simulink model "ssv_ssv_control"  (R2024a)
settings: Solver=VariableStepAuto  StartTime=0.0  StopTime=60.0  RelTol=1e-3
settings Model: Creator=MARTENAG  LastModifiedBy=MARTENAG

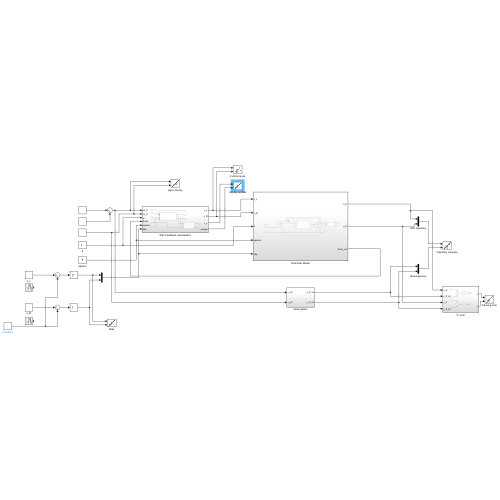
[thumbnail: Simulink's stored preview of the top-level diagram]
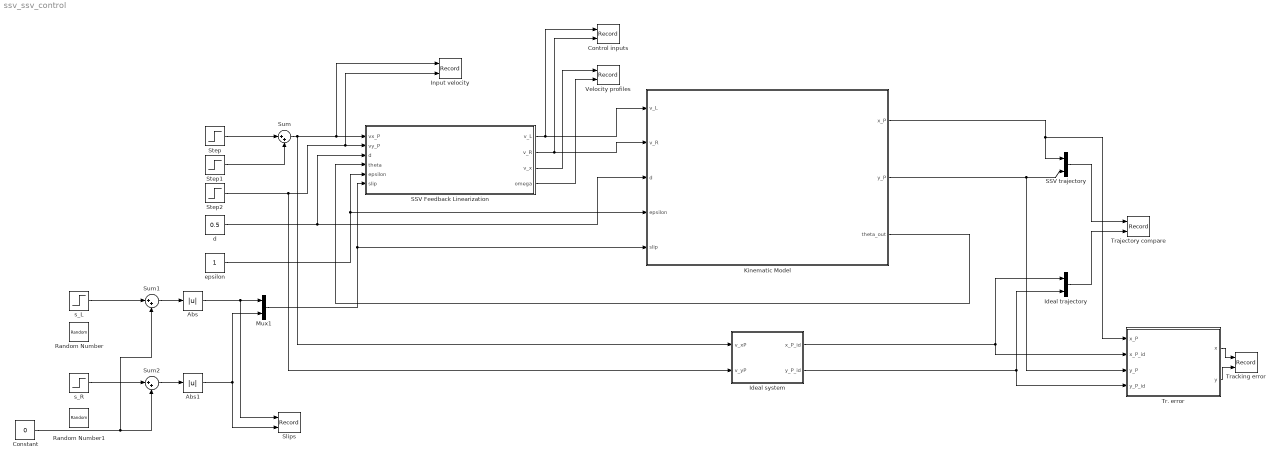
== system ssv_ssv_control ==
  Abs : Abs  SaturateOnIntegerOverflow=off
  Abs1 : Abs  SaturateOnIntegerOverflow=off
  Constant : Constant  Value=0
  Control inputs : Record  FileSettingsInternal="{\"entries\":[{\"content\":{\"excelSettings\":{\"content\":{},\"type\":\"Streamout.ExcelSettings\"}},\"type\":\"Streamout.FileSettingStorage\",\"uuid\":\"\"}],\"packageUris\":[\"http:\\/\\/schema.mathworks.com\\/mf0\\/streamout_blocks\\/R2020a\"],\"version\":\"1.0\"}"  Layout=[1 1]  SignalsInternal="{\"entries\":[{\"content\":{\"signals\":[{\"content\":{\"blockPath\":[],\"dimensions\":[1],\"domain\":\"\",\"lineColor\":\"#a2142f\",\"plots\":[ 1 ],\"port\":1,\"sid\":[\"\"],\"signalID\":1,\"signalName\":\"v_L\"},\"type\":\"RecordBlkView.Signal\",\"uuid\":\"\"},{\"content\":{\"blockPath\":[],\"dimensions\":[1],\"domain\":\"\",\"lineColor\":\"#139fff\",\"plots\":[ 1 ],\"port\":2,\"sid\":[\"\"],\"signalID\":2,\"signalName\":\"v_R\"},\"type\":\"RecordBlkView.Signal\",\"uuid\":\"\"}]},\"type\":\"RecordBlkView.InputSignals\",\"uuid\":\"\"}],\"packageUris\":[\"http:\\/\\/schema.mathworks.com\\/mf0\\/streamout_blocks\\/R2020a\"],\"version\":\"1.0\"}"  VisualizationBindings="{\"sparklinesplugin\":{\"info\":[{\"bindingParametersList\":[],\"subplotID\":1}]}}"  CompatibilityTag=XY
  Ideal system : Subsystem
  Ideal trajectory : Mux  Inputs=2
  Input velocity : Record  FileSettingsInternal="{\"entries\":[{\"content\":{\"excelSettings\":{\"content\":{},\"type\":\"Streamout.ExcelSettings\"}},\"type\":\"Streamout.FileSettingStorage\",\"uuid\":\"\"}],\"packageUris\":[\"http:\\/\\/schema.mathworks.com\\/mf0\\/streamout_blocks\\/R2020a\"],\"version\":\"1.0\"}"  Layout=[1 1]  SignalsInternal="{\"entries\":[{\"content\":{\"signals\":[{\"content\":{\"blockPath\":[],\"dimensions\":[1],\"domain\":\"\",\"lineColor\":\"#a2142f\",\"plots\":[ 1 ],\"port\":1,\"sid\":[\"\"],\"signalID\":1,\"signalName\":\"Sum\"},\"type\":\"RecordBlkView.Signal\",\"uuid\":\"\"},{\"content\":{\"blockPath\":[],\"dimensions\":[1],\"domain\":\"\",\"lineColor\":\"#139fff\",\"plots\":[ 1 ],\"port\":2,\"sid\":[\"\"],\"signalID\":2,\"signalName\":\"Step2\"},\"type\":\"RecordBlkView.Signal\",\"uuid\":\"\"}]},\"type\":\"RecordBlkView.InputSignals\",\"uuid\":\"\"}],\"packageUris\":[\"http:\\/\\/schema.mathworks.com\\/mf0\\/streamout_blocks\\/R2020a\"],\"version\":\"1.0\"}"  CompatibilityTag=XY
  Kinematic Model : Subsystem
  Mux1 : Mux  Inputs=2
  Random Number : RandomNumber  Mean=0.08  Variance=0.01  SampleTime=0.1
  Random Number1 : RandomNumber  Mean=0.08  Variance=0.01  SampleTime=0.1
  SSV Feedback Linearization : Subsystem
  SSV trajectory : Mux  Inputs=2
  Slips : Record  FileSettingsInternal="{\"entries\":[{\"content\":{\"excelSettings\":{\"content\":{},\"type\":\"Streamout.ExcelSettings\"}},\"type\":\"Streamout.FileSettingStorage\",\"uuid\":\"\"}],\"packageUris\":[\"http:\\/\\/schema.mathworks.com\\/mf0\\/streamout_blocks\\/R2020a\"],\"version\":\"1.0\"}"  Layout=[1 1]  SignalsInternal="{\"entries\":[{\"content\":{\"signals\":[{\"content\":{\"blockPath\":[],\"dimensions\":[1],\"domain\":\"\",\"lineColor\":\"#77ac30\",\"lineWidth\":2,\"plots\":[ 1 ],\"port\":1,\"sid\":[\"\"],\"signalID\":1,\"signalName\":\"Abs\"},\"type\":\"RecordBlkView.Signal\",\"uuid\":\"\"},{\"content\":{\"blockPath\":[],\"dimensions\":[1],\"domain\":\"\",\"lineColor\":\"#4dbeee\",\"lineWidth\":2,\"plots\":[ 1 ],\"port\":2,\"sid\":[\"\"],\"signalID\":2,\"signalName\":\"Abs1\"},\"type\":\"RecordBlkView.Signal\",\"uuid\":\"\"}]},\"type\":\"RecordBlkView.InputSignals\",\"uuid\":\"\"}],\"packageUris\":[\"http:\\/\\/schema.mathworks.com\\/mf0\\/streamout_blocks\\/R2020a\"],\"version\":\"1.0\"}"  VisualizationBindings="{\"sparklinesplugin\":{\"info\":[{\"bindingParametersList\":[],\"subplotID\":1}]}}"  CompatibilityTag=XY
  Step : Step  SampleTime=0
  Step1 : Step  Time=5  SampleTime=0
  Step2 : Step  Time=10  SampleTime=0
  Sum : Sum  Inputs=|++
  Sum1 : Sum  Inputs=|++
  Sum2 : Sum  Inputs=|++
  Tr. error : Subsystem
  Tracking error : Record  FileSettingsInternal="{\"entries\":[{\"content\":{\"excelSettings\":{\"content\":{},\"type\":\"Streamout.ExcelSettings\"}},\"type\":\"Streamout.FileSettingStorage\",\"uuid\":\"\"}],\"packageUris\":[\"http:\\/\\/schema.mathworks.com\\/mf0\\/streamout_blocks\\/R2020a\"],\"version\":\"1.0\"}"  Layout=[1 1]  SignalsInternal="{\"entries\":[{\"content\":{\"signals\":[{\"content\":{\"blockPath\":[],\"dimensions\":[1],\"domain\":\"\",\"lineColor\":\"#fe330a\",\"lineWidth\":2,\"plots\":[ 1 ],\"port\":1,\"sid\":[\"\"],\"signalID\":1,\"signalName\":\"Tr. error:1\"},\"type\":\"RecordBlkView.Signal\",\"uuid\":\"\"},{\"content\":{\"blockPath\":[],\"dimensions\":[1],\"domain\":\"\",\"lineColor\":\"#22b573\",\"lineWidth\":2,\"plots\":[ 1 ],\"port\":2,\"sid\":[\"\"],\"signalID\":2,\"signalName\":\"Tr. error:2\"},\"type\":\"RecordBlkView.Signal\",\"uuid\":\"\"}]},\"type\":\"RecordBlkView.InputSignals\",\"uuid\":\"\"}],\"packageUris\":[\"http:\\/\\/schema.mathworks.com\\/mf0\\/streamout_blocks\\/R2020a\"],\"version\":\"1.0\"}"  VisualizationBindings="{\"sparklinesplugin\":{\"info\":[{\"bindingParametersList\":[],\"subplotID\":1}]}}"  CompatibilityTag=XY
  Trajectory compare : Record  FileSettingsInternal="{\"entries\":[{\"content\":{\"excelSettings\":{\"content\":{},\"type\":\"Streamout.ExcelSettings\"}},\"type\":\"Streamout.FileSettingStorage\",\"uuid\":\"\"}],\"packageUris\":[\"http:\\/\\/schema.mathworks.com\\/mf0\\/streamout_blocks\\/R2020a\"],\"version\":\"1.0\"}"  Layout=[1 1]  SignalsInternal="{\"entries\":[{\"content\":{\"signals\":[{\"content\":{\"blockPath\":[],\"dimensions\":[2],\"domain\":\"\",\"hasChildren\":true,\"lineColor\":\"#77ac30\",\"lineWidth\":2,\"port\":1,\"sid\":[\"\"],\"signalID\":1,\"signalName\":\"SSV trajectory\"},\"type\":\"RecordBlkView.Signal\",\"uuid\":\"\"},{\"content\":{\"blockPath\":[],\"channel\":[1],\"dimensions\":[2],\"domain\":\"\",\"lineColor\":\"#139fff\",\"lineWidth\":2,\"parentID\":1,\"plots\":[ 1 ],\"port\":1,\"sid\":[\"\"],\"signalID\":2,\"signalName\":\"SSV trajectory\"},\"type\":\"RecordBlkView.Signal\",\"uuid\":\"\"},{\"content\":{\"blockPath\":[],\"dimensions\":[2],\"domain\":\"\",\"hasChildren\":true,\"lineColor\":\"#a2142f\",\"lineWidth\":2,\"port\":2,\"sid\":[\"\"],\"signalID\":3,\"signalName\":\"Ideal trajectory\"},\"type\":\"RecordBlkView.Signal\",\"uuid\":\"\"},{\"content\":{\"blockPath\":[],\"channel\":[1],\"dimensions\":[2],\"domain\":\"\",\"lineColor\":\"#b746ff\",\"lineWidth\":2,\"parentID\":3,\"plots\":[ 1 ],\"port\":2,\"sid\":[\"\"],\"signalID\":4,\"signalName\":\"Ideal trajectory\"},\"type\":\"RecordBlkView.Signal\",\"uuid\":\"\"},{\"content\":{\"blockPath\":[],\"channel\":[2],\"dimensions\":[2],\"domain\":\"\",\"lineColor\":\"#64d413\",\"lineWidth\":2,\"parentID\":1,\"plots\":[ 1 ],\"port\":1,\"sid\":[\"\"],\"signalID\":5,\"signalName\":\"SSV trajectory\"},\"type\":\"RecordBlkView.Signal\",\"uuid\":\"\"},{\"content\":{\"blockPath\":[],\"channel\":[2],\"dimensions\":[2],\"domain\":\"\",\"lineColor\":\"#ff13a6\",\"lineWidth\":2,\"parentID\":3,\"plots\":[ 1 ],\"port\":2,\"sid\":[\"\"],\"signalID\":6,\"signalName\":\"Ideal trajectory\"},\"type\":\"RecordBlkView.Signal\",\"uuid\":\"\"}]},\"type\":\"RecordBlkView.InputSignals\",\"uuid\":\"\"}],\"packageUris\":[\"http:\\/\\/schema.mathworks.com\\/mf0\\/streamout_blocks\\/R2020a\"],\"version\":\"1.0\"}"  VisualizationBindings="{\"xyplotplugin\":{\"info\":[{\"series\":[{\"bindingParametersList\":[{\"parameter\":\"X-Axis\",\"signalID\":4,\"signalName\":\"Ideal trajectory(1)\"},{\"parameter\":\"Y-Axis\",\"signalID\":6,\"signalName\":\"Ideal trajectory(2)\"}],\"seriesID\":0},{\"bindingParametersList\":[{\"parameter\":\"X-Axis\",\"signalID\":2,\"signalName\":\"SSV trajectory(1)\"},{\"parameter\":\"Y-Axis\",\"signalID\":5,\"signalName\":\"SSV trajectory(2)\"}],\"seriesID\":1}],\"subplotID\":1}]}}"  CompatibilityTag=XY
  Velocity profiles : Record  FileSettingsInternal="{\"entries\":[{\"content\":{\"excelSettings\":{\"content\":{},\"type\":\"Streamout.ExcelSettings\"}},\"type\":\"Streamout.FileSettingStorage\",\"uuid\":\"\"}],\"packageUris\":[\"http:\\/\\/schema.mathworks.com\\/mf0\\/streamout_blocks\\/R2020a\"],\"version\":\"1.0\"}"  Layout=[1 1]  SignalsInternal="{\"entries\":[{\"content\":{\"signals\":[{\"content\":{\"blockPath\":[],\"dimensions\":[1],\"domain\":\"\",\"lineColor\":\"#a2142f\",\"plots\":[ 1 ],\"port\":1,\"sid\":[\"\"],\"signalID\":1,\"signalName\":\"v_x\"},\"type\":\"RecordBlkView.Signal\",\"uuid\":\"\"},{\"content\":{\"blockPath\":[],\"dimensions\":[1],\"domain\":\"\",\"lineColor\":\"#139fff\",\"plots\":[ 1 ],\"port\":2,\"sid\":[\"\"],\"signalID\":2,\"signalName\":\"omega\"},\"type\":\"RecordBlkView.Signal\",\"uuid\":\"\"}]},\"type\":\"RecordBlkView.InputSignals\",\"uuid\":\"\"}],\"packageUris\":[\"http:\\/\\/schema.mathworks.com\\/mf0\\/streamout_blocks\\/R2020a\"],\"version\":\"1.0\"}"  VisualizationBindings="{\"sparklinesplugin\":{\"info\":[{\"bindingParametersList\":[],\"subplotID\":1}]}}"  CompatibilityTag=XY
  d : Constant  Value=0.5
  epsilon : Constant
  s_L : Step  Time=30  Before=0.05  After=0.1  SampleTime=0
  s_R : Step  Time=30  Before=0.05  After=0.25  SampleTime=0
  wires:
  Tr. error/1(x) -> Tracking error/1
  Ideal system/2(y_P_id) -> Tr. error/4(y_P_id), Ideal trajectory/2
  Ideal system/1(x_P_id) -> Tr. error/2(x_P_id), Ideal trajectory/1
  Kinematic Model/3(theta_out) -> SSV Feedback Linearization/4(theta)
  Kinematic Model/1(x_P) -> SSV trajectory/1, Tr. error/1(x_P)
  Tr. error/2(y) -> Tracking error/2
  Kinematic Model/2(y_P) -> Tr. error/3(y_P), SSV trajectory/2
  Ideal trajectory/1 -> Trajectory compare/2
  SSV trajectory/1 -> Trajectory compare/1
  Step2/1 -> SSV Feedback Linearization/2(vy_P), Input velocity/2, Ideal system/2(v_yP)
  Sum/1 -> Input velocity/1, SSV Feedback Linearization/1(vx_P), Ideal system/1(v_xP)
  Step1/1 -> Sum/2
  d/1 -> SSV Feedback Linearization/3(d), Kinematic Model/3(d)
  epsilon/1 -> SSV Feedback Linearization/5(epsilon), Kinematic Model/4(epsilon)
  Step/1 -> Sum/1
  Mux1/1 -> Kinematic Model/5(slip), SSV Feedback Linearization/6(slip)
  SSV Feedback Linearization/1(v_L) -> Control inputs/1, Kinematic Model/1(v_L)
  SSV Feedback Linearization/2(v_R) -> Control inputs/2, Kinematic Model/2(v_R)
  SSV Feedback Linearization/3(v_x) -> Velocity profiles/1
  SSV Feedback Linearization/4(omega) -> Velocity profiles/2
  s_L/1 -> Sum1/1
  Sum2/1 -> Abs1/1
  Sum1/1 -> Abs/1
  s_R/1 -> Sum2/1
  Abs/1 -> Slips/1, Mux1/1
  Abs1/1 -> Slips/2, Mux1/2
  Constant/1 -> Sum1/2, Sum2/2

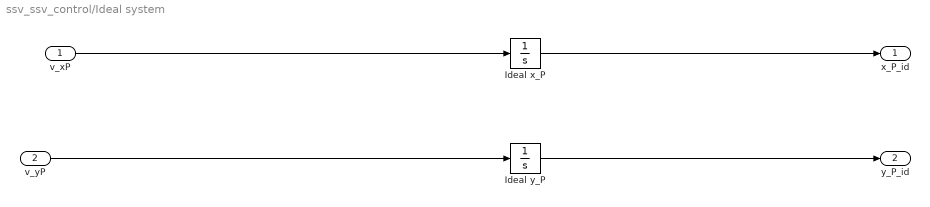
== system ssv_ssv_control/Ideal system ==
  v_xP : Inport
  v_yP : Inport  Port=2
  Ideal x_P : Integrator
  Ideal y_P : Integrator
  x_P_id : Outport
  y_P_id : Outport  Port=2
  wires:
  Ideal x_P/1 -> x_P_id/1
  Ideal y_P/1 -> y_P_id/1
  v_yP/1 -> Ideal y_P/1
  v_xP/1 -> Ideal x_P/1

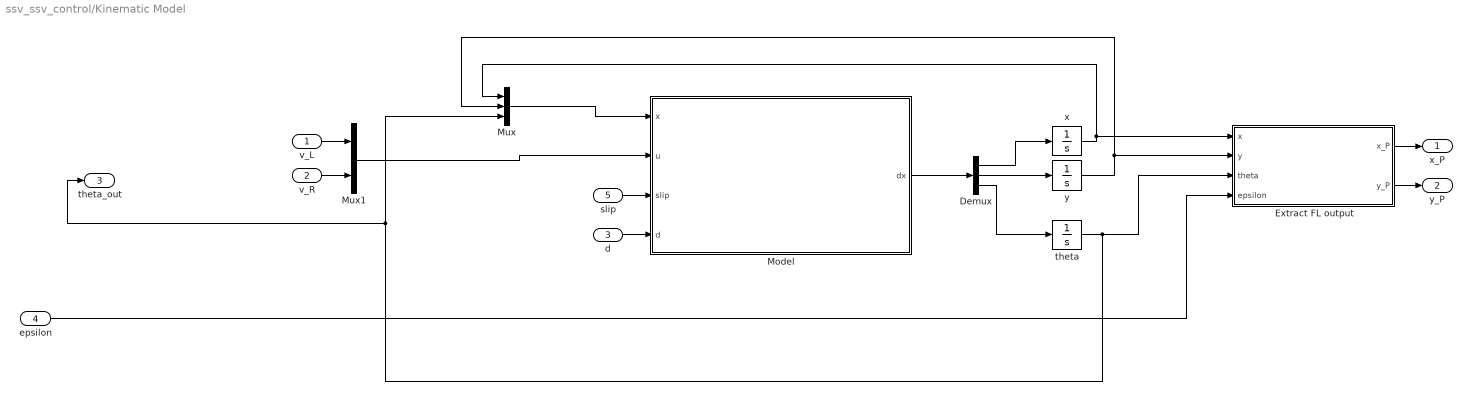
== system ssv_ssv_control/Kinematic Model ==
  v_L : Inport
  v_R : Inport  Port=2
  d : Inport  Port=3
  epsilon : Inport  Port=4
  slip : Inport  Port=5
  Demux : Demux  Outputs=3
  Extract FL output : MATLAB Function  TreatAsAtomicUnit=on
  Model : MATLAB Function  TreatAsAtomicUnit=on
  Mux : Mux  Inputs=3
  Mux1 : Mux  Inputs=2
  theta : Integrator
  x : Integrator
  y : Integrator
  x_P : Outport
  y_P : Outport  Port=2
  theta_out : Outport  Port=3
  wires:
  Demux/2 -> y/1
  x/1 -> Mux/1, Extract FL output/1(x)
  Mux1/1 -> Model/2(u)
  Mux/1 -> Model/1(x)
  d/1 -> Model/4(d)
  epsilon/1 -> Extract FL output/4(epsilon)
  Model/1(dx) -> Demux/1
  Demux/1 -> x/1
  theta/1 -> Extract FL output/3(theta), theta_out/1, Mux/3
  Demux/3 -> theta/1
  y/1 -> Extract FL output/2(y), Mux/2
  Extract FL output/1(x_P) -> x_P/1
  v_L/1 -> Mux1/1
  v_R/1 -> Mux1/2
  Extract FL output/2(y_P) -> y_P/1
  slip/1 -> Model/3(slip)

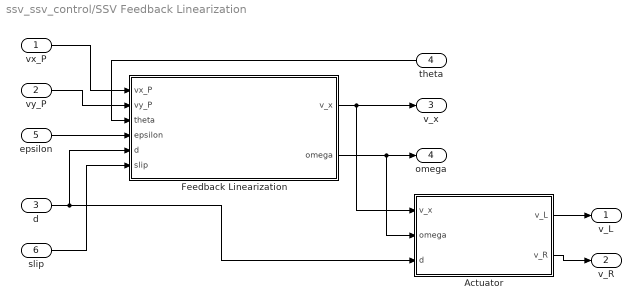
== system ssv_ssv_control/SSV Feedback Linearization ==
  vx_P : Inport
  vy_P : Inport  Port=2
  d : Inport  Port=3
  theta : Inport  Port=4
  epsilon : Inport  Port=5
  slip : Inport  Port=6
  Actuator : MATLAB Function  TreatAsAtomicUnit=on
  Feedback Linearization : MATLAB Function  TreatAsAtomicUnit=on
  v_L : Outport
  v_R : Outport  Port=2
  v_x : Outport  Port=3
  omega : Outport  Port=4
  wires:
  vx_P/1 -> Feedback Linearization/1(vx_P)
  vy_P/1 -> Feedback Linearization/2(vy_P)
  theta/1 -> Feedback Linearization/3(theta)
  slip/1 -> Feedback Linearization/6(slip)
  d/1 -> Actuator/3(d), Feedback Linearization/5(d)
  epsilon/1 -> Feedback Linearization/4(epsilon)
  Feedback Linearization/2(omega) -> omega/1, Actuator/2(omega)
  Feedback Linearization/1(v_x) -> Actuator/1(v_x), v_x/1
  Actuator/1(v_L) -> v_L/1
  Actuator/2(v_R) -> v_R/1

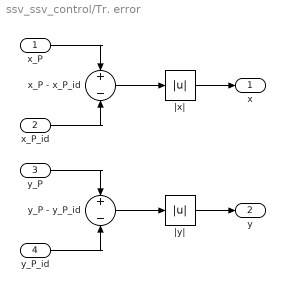
== system ssv_ssv_control/Tr. error ==
  x_P : Inport
  x_P_id : Inport  Port=2
  y_P : Inport  Port=3
  y_P_id : Inport  Port=4
  x_P - x_P_id : Sum  Inputs=+-
  y_P - y_P_id : Sum  Inputs=+-
  |x| : Abs  SaturateOnIntegerOverflow=off
  |y| : Abs  SaturateOnIntegerOverflow=off
  x : Outport
  y : Outport  Port=2
  wires:
  |y|/1 -> y/1
  y_P - y_P_id/1 -> |y|/1
  x_P - x_P_id/1 -> |x|/1
  y_P_id/1 -> y_P - y_P_id/2
  y_P/1 -> y_P - y_P_id/1
  x_P_id/1 -> x_P - x_P_id/2
  x_P/1 -> x_P - x_P_id/1
  |x|/1 -> x/1

== matlab function ssv_ssv_control/SSV Feedback Linearization/Actuator ==
  data: v_x input; v_L output; omega input; d input; v_R output
function [v_L, v_R] = actuator(v_x, omega, d)
    v_L = v_x - d*omega;
    v_R = v_x + d*omega;
end

== matlab function ssv_ssv_control/Kinematic Model/Model ==
  data: x input size=3; dx output size=3; u input size=2; slip input size=2; d input size=1
function dx = kinematic_model(x, u, slip, d)
% Inputs:
    % x = [x; y; theta] (state vector)
    % u = [v_L; v_R] (control inputs: left and right wheel velocities)
    % slip = [s_L; s_R] (slip coefficients for left and right wheels)
    % d (half the track width)
    
    % Extract slip
    s_L = slip(1);
    s_R = slip(2);

    % Extract state variables
    theta = x(3);

    % Extract control inputs
    v_L = u(1);
    v_R = u(2);
    
    % Kinematic equations
    dx = zeros(3,1);
    dx(1) = ((1-s_R)/2 * cos(theta) * v_R) + ((1-s_L)/2 * cos(theta) * v_L);
    dx(2) = ((1-s_R)/2 * sin(theta) * v_R) + ((1-s_L)/2 * sin(theta) * v_L);
    dx(3) = (1-s_R)/(2*d)*v_R - (1-s_L)/(2*d)*v_L;
end

== matlab function ssv_ssv_control/SSV Feedback Linearization/Feedback Linearization ==
  data: vx_P input; v_x output; vy_P input; theta input; epsilon input; d input; slip input; omega output
function [v_x, omega] = ssv_feedback_linearization(vx_P, vy_P, theta, epsilon, d, slip)
    s_L = slip(1);
    s_R = slip(2);

    eta_L = 1 - s_L;
    eta_R = 1 - s_R;
    gamma_11 = (eta_L + eta_R) / 2;
    gamma_12 = (eta_L - eta_R) / 2;
    gamma_21 = (eta_L + eta_R) / d;
    gamma_22 = (eta_L - eta_R) / d;

    v_x = 1 / (epsilon*eta_L*eta_R) * ((epsilon*gamma_11*cos(theta)-d*gamma_12*sin(theta)) * vx_P + (epsilon*gamma_11*sin(theta)+d*gamma_12*cos(theta)) * vy_P);
    omega = 1 / (epsilon*eta_L*eta_R) * ((epsilon*gamma_22*cos(theta)-d*gamma_21*sin(theta)) * vx_P + (epsilon*gamma_22*sin(theta)+d*gamma_21*cos(theta)) * vy_P);
end

== matlab function ssv_ssv_control/Kinematic Model/Extract FL output ==
  data: x input; x_P output; y input; theta input; epsilon input; y_P output
function [x_P, y_P] = extract_fl_output(x, y, theta, epsilon)
    x_P = x + epsilon*cos(theta);
    y_P = y + epsilon*sin(theta);
end
